simulink model "Simulink_MPC_LQR"  (R2025b)
settings: Solver=VariableStepAuto  StartTime=0.0  StopTime=50  RelTol=1e-3
InitFcn:
  | run("init.m");
StopFcn:
  | %run("video.m");
undefined symbols (not defined in the file or in its folder): robot_params
settings Model: Creator=Acer  LastModifiedBy=Acer

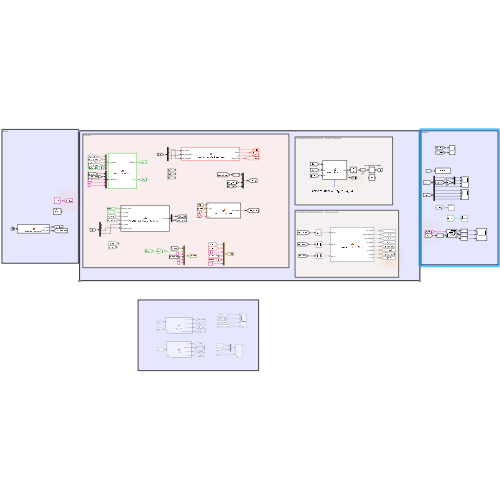
[thumbnail: Simulink's stored preview of the top-level diagram]
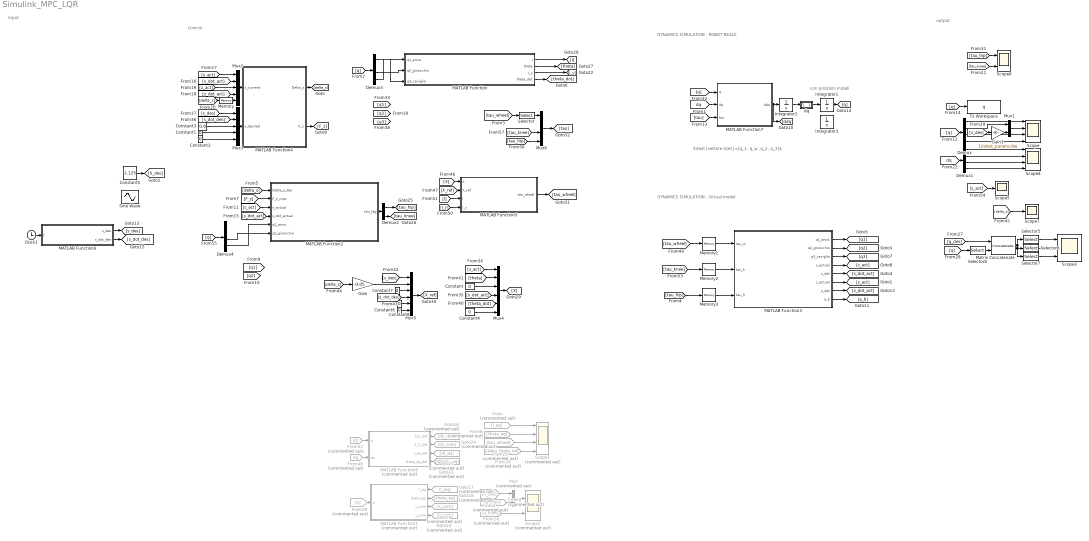
== system Simulink_MPC_LQR ==
  note: con posizioni iniziali
  note: input
  note: output
  note: DYNAMICS SIMULATION - ROBOT REALE
  note: $\text{vettore stati}=[q_1, q_w ,q_2, q_3]$
  note: Control
  note: DYNAMICS SIMULATION - Virtual model
  Clock1 : Clock
  Constant{,1..2,4,6..8} (7 alike) : Constant  Value=0
  Constant3 : Constant  Value=0.6
  Constant5 : Constant  Value=1.125
  Demux{,1,3..4} (4 alike) : Demux
  Demux2 : Demux  Outputs=2
  From : From  Commented=on  GotoTag=l_eq
  From23 : From  Commented=on  GotoTag=h_des
  From24 : From  Commented=on  GotoTag=s_com
  From25 : From  Commented=on  GotoTag=tau_wheel
  From26 : From  Commented=on  GotoTag=delta_theta_ref
  From39 : From  Commented=on  GotoTag=q
  From48 : From  Commented=on  GotoTag=dq  TagVisibility=global
  From52 : From  Commented=on  GotoTag=q
  From6 : From  Commented=on  GotoTag=theta_eq
  From8 : From  Commented=on  GotoTag=z_com
  Gain : Gain  Gain=-0.05
  Gain3 : Gain  Gain=1/robot_params.Rw
  Goto16 : Goto  Commented=on  GotoTag=ds_com
  Goto17 : Goto  Commented=on  GotoTag=l_eq
  Goto18 : Goto  Commented=on  GotoTag=theta_eq
  Goto19 : Goto  Commented=on  GotoTag=s_com
  Goto20 : Goto  Commented=on  GotoTag=z_com
  Goto21 : Goto  Commented=on  GotoTag=dl_eq
  Goto23 : Goto  Commented=on  GotoTag=dtheta_eq
  Goto24 : Goto  Commented=on  GotoTag=dz_com
  Integrator1 : Integrator  InitialCondition=[2.68;0;-2.34;1.23]
  Integrator2 : Integrator  InitialCondition=zeros(4,1)
  Integrator3 : Integrator  InitialCondition=[pi/2-0.1;zeros(3,1)]
  MATLAB Function : MATLAB Function  TreatAsAtomicUnit=on
  MATLAB Function1 : MATLAB Function  Commented=on  TreatAsAtomicUnit=on
  MATLAB Function2 : MATLAB Function  TreatAsAtomicUnit=on
  MATLAB Function3 : MATLAB Function  TreatAsAtomicUnit=on
  MATLAB Function4 : MATLAB Function  TreatAsAtomicUnit=on
  MATLAB Function5 : MATLAB Function  TreatAsAtomicUnit=on
  MATLAB Function6 : MATLAB Function  TreatAsAtomicUnit=on
  MATLAB Function7 : MATLAB Function  TreatAsAtomicUnit=on
  MATLAB Function8 : MATLAB Function  Commented=on  TreatAsAtomicUnit=on
  Matrix Concatenate : Concatenate  Mode=Multidimensional array  ConcatenateDimension=2
  Memory{,1..3} (4 alike) : Memory
  Mux : Mux  Commented=on  Inputs=2
  Mux1 : Mux  Inputs=2
  Mux2 : Mux  Inputs=5
  Mux3 : Mux  Inputs=5
  Mux4 : Mux  Inputs=6
  Mux5 : Mux  Inputs=6
  Mux6 : Mux
  Scope : Scope  NumInputPorts=4
      settings: ActiveDisplayString=4  Title=q3  ActiveDisplayYMinimum=-65.728095745464827  ActiveDisplayYMaximum=20.305803066962241
  Scope1 : Scope  Commented=on  NumInputPorts=4
      settings: ActiveDisplayString=4  Title=Delta_theta_ref  ActiveDisplayYMinimum=-0.047873246159911287  ActiveDisplayYMaximum=0.27907655031491813
  Scope2 : Scope  Commented=on  NumInputPorts=2
      settings: ActiveDisplayYMinimum=0.29186136198287116  ActiveDisplayYMaximum=1.3009042931130141  DataLoggingVariableName=ScopeData2
  Scope3 : Scope  NumInputPorts=3
      settings: ActiveDisplayYMinimum=2.02772604544463  ActiveDisplayYMaximum=2.8223539236982456  DataLoggingVariableName=ScopeData3
  Scope4 : Scope  NumInputPorts=4
      settings: Title=dq1  ActiveDisplayYMinimum=-1.1906100272021516  ActiveDisplayYMaximum=1.6920979215580041  DataLoggingVariableName=ScopeData4
  Scope5 : Scope
      settings: ActiveDisplayYMinimum=-44.629750975469719  ActiveDisplayYMaximum=5.655822114795205  DataLoggingVariableName=ScopeData5
  Scope7 : Scope
      settings: ActiveDisplayYMinimum=-0.6644623531131485  ActiveDisplayYMaximum=2.1105376468868529  DataLoggingVariableName=ScopeData7
  Scope8 : Scope  NumInputPorts=2
      settings: ActiveDisplayYMinimum=-6.3705206521435818  ActiveDisplayYMaximum=7.5706457083104626  DataLoggingVariableName=ScopeData8
  Selector : Selector  InputPortWidth=2  IndexOptions=Index vector (dialog)  Indices=1  OutputSizes=1
  Selector5 : Selector  NumberOfDimensions=2  InputPortWidth=3  IndexOptions=Index vector (dialog),Index vector (dialog)  Indices=[1],[1 2]  OutputSizes=1,1
  Selector6 : Selector  NumberOfDimensions=2  InputPortWidth=3  IndexOptions=Index vector (dialog),Index vector (dialog)  Indices=[2],[1 2]  OutputSizes=1,1
  Selector7 : Selector  NumberOfDimensions=2  InputPortWidth=3  IndexOptions=Index vector (dialog),Index vector (dialog)  Indices=[3],[1 2]  OutputSizes=1,1
  Selector8 : Selector  InputPortWidth=4  IndexOptions=Index vector (dialog)  Indices=[1 3 4]  OutputSizes=1
  Sine Wave : Sin  Amplitude=0.1  Bias=0.7  SampleTime=0
  To Workspace : ToWorkspace  VariableName=q  SaveFormat=Timeseries  SampleTime=-1
  dq : Subsystem
  wires:
  [tau] -> MATLAB Function7/3(tau)
  [q] -> MATLAB Function7/1(q)
  Integrator1/1 -> [q]
  MATLAB Function7/1(ddq) -> [ddq], Integrator2/1
  [dq] -> MATLAB Function7/2(dq)
  Integrator2/1 -> dq/1(In1)
  dq/1(Out1) -> Integrator1/1
  Demux/1 -> Scope/1
  Demux/3 -> Scope/3
  Demux/4 -> Scope/4
  [q] -> Demux/1
  [q] -> To Workspace/1
  MATLAB Function1/4(z_com) -> Goto20/1
  MATLAB Function8/2(Z_C_dot) -> Goto24/1
  MATLAB Function1/3(s_com) -> Goto19/1
  MATLAB Function8/4(theta_eq_dot) -> Goto23/1
  MATLAB Function1/1(l_eq) -> Goto17/1
  From52/1 -> MATLAB Function8/1(q)
  From39/1 -> MATLAB Function1/1(q)
  MATLAB Function1/2(theta_eq) -> Goto18/1
  MATLAB Function8/3(l_eq_dot) -> Goto21/1
  From48/1 -> MATLAB Function8/2(dq)
  MATLAB Function8/1(S_C_dot) -> Goto16/1
  From/1 -> Scope1/1
  From6/1 -> Scope1/2
  Constant5/1 -> [h_des]
  From8/1 -> Mux/2
  From23/1 -> Mux/1
  From24/1 -> Scope2/2
  Mux/1 -> Scope2/1
  [q_des] -> Matrix Concatenate/1
  Matrix Concatenate/1 -> Selector7/1, Selector6/1, Selector5/1
  Selector5/1 -> Scope3/1
  Selector6/1 -> Scope3/2
  Selector7/1 -> Scope3/3
  [q] -> Selector8/1
  Selector8/1 -> Matrix Concatenate/2
  From25/1 -> Scope1/3
  From26/1 -> Scope1/4
  Demux1/4 -> Scope4/4
  Demux1/3 -> Scope4/3
  Demux1/1 -> Scope4/1
  Demux1/2 -> Scope4/2
  [dq] -> Demux1/1
  [s_des] -> Gain3/1
  Mux1/1 -> Scope/2
  Demux/2 -> Mux1/1
  Gain3/1 -> Mux1/2
  MATLAB Function3/2(q2_ginocchio) -> [q2]
  MATLAB Function3/7(z_dot) -> [z_dot_act]
  Memory2/1 -> MATLAB Function3/2(tau_k)
  MATLAB Function3/3(q3_caviglia) -> [q3]
  [tau_knee] -> Memory2/1
  MATLAB Function3/8(a_b) -> [a_b]
  MATLAB Function3/1(q1_anca) -> [q1]
  MATLAB Function3/4(s_actual) -> [s_act]
  Memory3/1 -> MATLAB Function3/3(tau_h)
  [tau_hip] -> Memory3/1
  MATLAB Function3/5(s_dot) -> [s_dot_act]
  MATLAB Function3/6(z_actual) -> [z_act]
  Memory1/1 -> MATLAB Function3/1(tau_w)
  [tau_wheel] -> Memory1/1
  [s_dot_act] -> Mux2/2
  Memory/1 -> Mux2/5
  [z_dot_act] -> Mux2/4
  [s_act] -> Mux2/1
  [z_act] -> Mux2/3
  [delta_s] -> Memory/1
  Mux2/1 -> MATLAB Function4/1(x_current)
  MATLAB Function6/2(s_dot_des) -> [s_dot_des]
  Constant1/1 -> Mux3/4
  Constant3/1 -> Mux3/3
  Clock1/1 -> MATLAB Function6/1(t)
  MATLAB Function6/1(s_des) -> [s_des]
  Constant2/1 -> Mux3/5
  [s_des] -> Mux3/1
  [s_dot_des] -> Mux3/2
  Mux3/1 -> MATLAB Function4/2(x_desired)
  MATLAB Function4/1(Delta_s) -> [delta_s]
  MATLAB Function4/2(F_z) -> [F_z]
  [s_act] -> MATLAB Function2/3(s_actual)
  Demux4/3 -> MATLAB Function2/6(q2_ginocchio)
  [delta_s] -> MATLAB Function2/1(Delta_s_des)
  Demux4/4 -> MATLAB Function2/5(q1_anca)
  Demux2/1 -> [tau_hip]
  [F_z] -> MATLAB Function2/2(F_z_mpc)
  MATLAB Function2/1(tau_leg) -> Demux2/1
  [s_dot_act] -> MATLAB Function2/4(s_dot_actual)
  [tau_knee] -> Scope8/2
  [tau_hip] -> Scope8/1
  Demux2/2 -> [tau_knee]
  Demux3/3 -> MATLAB Function/2(q2_ginocchio)
  Demux3/1 -> MATLAB Function/3(q3_caviglia)
  Demux3/4 -> MATLAB Function/1(q1_anca)
  MATLAB Function/4(theta_dot) -> [theta_dot]
  MATLAB Function/3(I_y) -> [I_y]
  MATLAB Function/1(l) -> [l]
  MATLAB Function/2(theta) -> [theta]
  [s_act] -> Mux4/1
  [s_dot_act] -> Mux4/4
  [theta_dot] -> Mux4/5
  [theta] -> Mux4/2
  Constant/1 -> Mux4/3
  Constant4/1 -> Mux4/6
  Mux4/1 -> [X]
  Gain/1 -> Mux5/2
  [delta_s] -> Gain/1
  Mux5/1 -> [X_ref]
  [s_dot_des] -> Mux5/4
  [s_des] -> Mux5/1
  [delta_s] -> Scope7/1
  Constant7/1 -> Mux5/3
  Constant8/1 -> Mux5/5
  Constant6/1 -> Mux5/6
  [X] -> MATLAB Function5/1(X)
  [X_ref] -> MATLAB Function5/2(X_ref)
  [I_y] -> MATLAB Function5/4(I_y)
  [l] -> MATLAB Function5/3(l)
  MATLAB Function5/1(tau_wheel) -> [tau_wheel]
  [q] -> Demux3/1
  [s_act] -> Scope5/1
  [q] -> Demux4/1
  Mux6/1 -> [tau]
  [tau_knee] -> Mux6/3
  [tau_hip] -> Mux6/4
  [tau_wheel] -> Selector/1
  Selector/1 -> Mux6/1

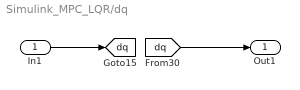
== system Simulink_MPC_LQR/dq ==
  In1 : Inport
  Out1 : Outport
  tag scope: dq=global
  wires:
  In1/1 -> [dq]
  [dq] -> Out1/1

== matlab function Simulink_MPC_LQR/MATLAB Function8 ==
  data: q input; dq input; S_C_dot output; Z_C_dot output; l_eq_dot output; theta_eq_dot output; robot_params parameter
function [S_C_dot, Z_C_dot, l_eq_dot, theta_eq_dot] = J_CoM(q,dq,robot_params)
    %#codegen
    % CALCOLA_VELOCITA_COM_SIMULINK Calcola le velocità del CoM e del pendolo 
    % equivalente (WIP) per l'utilizzo in Simulink.
    
    % --- 1. Estrazione Variabili di Stato ---
    q1 = q(1);
    q2 = q(3);
    q3 = q(4);
    
    % --- 2. Estrazione Parametri Robot ---
    l1 = robot_params.l1;
    l2 = robot_params.l2;
    l3 = robot_params.l3;
    
    m1 = robot_params.m1;
    m2 = robot_params.m2;
    m3 = robot_params.m3;
    m_upper = m1 + m2 + m3;
    
    % --- 3. Costanti Raggruppate per l'Analitica ---
    K1 = (m1 * (l1/2) + m2 * l1 + m3 * l1) / m_upper;
    K2 = (m2 * (l2/2) + m3 * l2) / m_upper;
    K3 = (m3 * (l3/2)) / m_upper;
    
    % --- 4. Ricalcolo Posizione CoM ---
    S_C = K1*cos(q1) + K2*cos(q1+q2) + K3*sin(q3);
    Z_C = K1*sin(q1) + K2*sin(q1+q2) + K3*cos(q3);
    
    % --- 5. Calcolo Jacobiano (J_CoM) ---
    % Preallocazione statica della matrice 2x4 per compatibilità C/C++
    J_CoM = zeros(2, 4);
    
   % --- 5. Calcolo Jacobiano (J_CoM) ---
    % Preallocazione statica della matrice 2x4 per compatibilità C/C++
    J_CoM = zeros(2, 4);
    
    % Derivate parziali di S_C (Prima Riga)
    J_CoM(1, 1) = -K1*sin(q1) - K2*sin(q1+q2); % <--- CORRETTO: indice (1,1) per dq1
    J_CoM(1, 3) = -K2*sin(q1+q2);              % <--- CORRETTO: indice (1,3) per dq2
    J_CoM(1, 4) =  K3*cos(q3);                 % <--- CORRETTO: indice (1,4) per dq3
    
    % Derivate parziali di Z_C (Seconda Riga)
    J_CoM(2, 1) =  K1*cos(q1) + K2*cos(q1+q2); % <--- CORRETTO: indice (2,1) per dq1
    J_CoM(2, 3) =  K2*cos(q1+q2);              % <--- CORRETTO: indice (2,3) per dq2
    J_CoM(2, 4) = -K3*sin(q3);                 % <--- CORRETTO: indice (2,4) per dq3
    % --- 6. Calcolo Velocità Cartesiane ---
    % V_C = [S_C_dot; Z_C_dot]
    V_C = J_CoM * dq;
    S_C_dot = V_C(1);
    Z_C_dot = V_C(2);
    
    % --- 7. Derivate del Pendolo Equivalente e Gestione Singolarità ---
    l_eq_sq = S_C^2 + Z_C^2;
    l_eq = sqrt(l_eq_sq);
    

        l_eq_dot = (S_C * S_C_dot + Z_C * Z_C_dot) / l_eq;
        theta_eq_dot = (S_C_dot * Z_C - S_C * Z_C_dot) / l_eq_sq;
   end

== matlab function Simulink_MPC_LQR/MATLAB Function ==
  settings: updateMethod=DISCRETE  sampleTime=0.001
  data: q1_anca input; l output; q2_ginocchio input; q3_caviglia input; theta output; I_y output; theta_dot output
function [l, theta, I_y, theta_dot] = calculate_equivalent_pendulum(q1_anca, q2_ginocchio, q3_caviglia)
    persistent theta_prev
    if isempty(theta_prev), theta_prev = 0; end
    dt = 0.001;

    % Somma degli angoli della catena
    theta = q1_anca + q2_ginocchio + q3_caviglia;
    theta_dot = (theta - theta_prev) / dt;
    theta_prev = theta;

    l = 2 * 0.45 * cos(q2_ginocchio / 2);
    if l < 0.1, l = 0.1; end
    m_b = 73.0;
    I_y = (1/3) * m_b * l^2;
end

== matlab function Simulink_MPC_LQR/MATLAB Function3 ==
  data: tau_w input; q1_anca output; tau_k input; tau_h input; q2_ginocchio output; q3_caviglia output; s_actual output; s_dot output; z_actual output; z_dot output; a_b output
function [q1_anca, q2_ginocchio, q3_caviglia, s_actual, s_dot, z_actual, z_dot, a_b] = Simulated_Robot_Plant(tau_w, tau_k, tau_h)
    q1_anca = 0.0; q2_ginocchio = 0.0; q3_caviglia = 0.0;
    s_actual = 0.0; s_dot = 0.0; z_actual = 0.0; z_dot = 0.0;
    a_b = zeros(2,1);

    persistent X_z X_wip
    if isempty(X_z)
        X_z = [0.6; 0];       
        X_wip = [0; 0; 0; 0]; 
    end
    dt = 0.001; g = 9.81; m_b = 73.0; r = 0.127; m_w = 3.5; I_w = 0.1; l = 0.45;

    %% 1. FISICA VERTICALE (Z)
    ratio = X_z(1) / (2*l);
    if ratio > 0.999, ratio = 0.999; elseif ratio < -0.999, ratio = -0.999; end
    q2_current = 2 * acos(ratio);
    
    J_z_knee = -l * sin(q2_current / 2);
    if abs(J_z_knee) < 0.05, J_z_knee = -0.05 * sign(q2_current + 1e-6); end
    
    F_z_applied = tau_k / J_z_knee; 
    z_ddot = (F_z_applied / m_b) - g;
    
    X_z(2) = X_z(2) + z_ddot * dt;
    X_z(1) = X_z(1) + X_z(2) * dt;
    
    % Blocchi fisici estremi per evitare decolli o sprofondamenti
    if X_z(1) < 0.2, X_z(1) = 0.2; X_z(2) = 0; end 
    if X_z(1) > 0.9, X_z(1) = 0.9; X_z(2) = 0; end 
    z_act = X_z(1);

    %% 2. FISICA DEL PENDOLO Orizzontale
    l_pend = z_act;
    if l_pend > 0.9, l_pend = 0.9; end 
    if l_pend < 0.1, l_pend = 0.1; end
    
    I_y = (1/3) * m_b * l_pend^2;

    D = 2*I_w*(I_y + m_b*l_pend^2) + (2*l_pend^2*m_b*m_w + I_y*(m_b + 2*m_w)*r^2);
    a1 = -(g * l_pend^2 * m_b^2 * r^2) / D;
    a2 =  (g * l_pend * m_b * (2*I_w + (m_b + 2*m_w)*r^2)) / D;
    b1 =  (r * (I_y + l_pend*m_b*(l_pend + r))) / D;
    b2 = -(2*I_w + r*(l_pend*m_b + (m_b + 2*m_w)*r)) / D;

    A_wip = [0 0 1 0; 0 0 0 1; 0 a1 0 0; 0 a2 0 0];
    B_wip = [0 0; 0 0; b1 b1; b2 b2];

    % LA CORREZIONE VITALE: Diamo ai motori la forza di bilanciare 73 kg!
    tau_w_lim = tau_w;
    limite = 1000; % Aumentato da 15 a 1000 Nm
    if tau_w_lim(1) > limite, tau_w_lim(1) = limite; end
    if tau_w_lim(1) < -limite, tau_w_lim(1) = -limite; end
    if tau_w_lim(2) > limite, tau_w_lim(2) = limite; end
    if tau_w_lim(2) < -limite, tau_w_lim(2) = -limite; end

    X_wip_dot = A_wip * X_wip + B_wip * tau_w_lim;
    X_wip = X_wip + X_wip_dot * dt;
    theta_vero = X_wip(2);

    %% 3. ASSEGNAZIONE GIUNTI (La tua convenzione perfetta)
    ratio_new = z_act / (2*l);
    if ratio_new > 0.999, ratio_new = 0.999; elseif ratio_new < -0.999, ratio_new = -0.999; end
    q2_ginocchio = 2 * acos(ratio_new);
    
    alpha = q2_ginocchio / 2;
    q3_caviglia = -alpha + theta_vero;
    q1_anca = -alpha;

    %% 4. ASSEGNAZIONE USCITE
    s_actual = X_wip(1);
    s_dot = X_wip(3);
    z_actual = z_act;
    z_dot = X_z(2);
    a_b = [X_wip_dot(3); z_ddot + g];
end

== matlab function Simulink_MPC_LQR/MATLAB Function6 ==
  data: t input; s_des output; s_dot_des output
function [s_des, s_dot_des] = Smooth_Trajectory(t)
    % PRE-ALLOCAZIONE PER IL CODER
    s_des = 0.0;
    s_dot_des = 0.0;
    
    % PARAMETRI DELLA TRAIETTORIA
    t_start = 0.0;       % Il robot inizia a muoversi a 2 secondi
    t_end = 5.0;         % Arriva a destinazione a 5 secondi (3 secondi di viaggio)
    s_final = 1.0;       % Destinazione orizzontale (1 metro)
    
    % LOGICA DEL MOVIMENTO
    if t <= t_start
        % Prima di partire, resta fermo
        s_des = 0.0;
        s_dot_des = 0.0;
        
    elseif t >= t_end
        % Arrivato a destinazione, fermati
        s_des = s_final;
        s_dot_des = 0.0;
        
    else
        % FASE DI MOTO: Polinomio Cubico (Minimum Jerk Trajectory)
        % Normalizziamo il tempo tra 0 e 1 per la durata del viaggio
        tau = (t - t_start) / (t_end - t_start);
        
        % Posizione (Profilo a "S" morbida)
        s_des = s_final * (3*tau^2 - 2*tau^3);
        
        % Velocità (Derivata della posizione, forma a campana)
        s_dot_des = s_final * (6*tau - 6*tau^2) / (t_end - t_start);
    end
end

== matlab function Simulink_MPC_LQR/MATLAB Function4 ==
  settings: updateMethod=DISCRETE  sampleTime=0.01
  data: x_current input; Delta_s output; x_desired input; F_z output
function [Delta_s,F_z] = MPC_Custom_QP(x_current, x_desired)
    % quadprog non è supportato nativamente per la code generation C
    coder.extrinsic('quadprog');
    coder.extrinsic('optimoptions');

    %% 1. Parametri e Discretizzazione
    m_b = 73.0; 
    g = 9.81;    
    
    h = x_current(3); 
    if h < 0.1
        h = 0.6;
    end
    
    dt = 0.01; 
    N = 40;     
    
    A_c = zeros(5,5);
    A_c(1,2) = 1;
    A_c(3,4) = 1;
    A_c(2,5) = g / h; 
    
    B_c = zeros(5,2);
    B_c(4,2) = 1 / m_b;
    B_c(5,1) = 1;
    
    A_d = eye(5) + A_c * dt;
    B_d = B_c * dt;

    %% 2. Pesi della Funzione di Costo
    S = diag([100, 10, 500, 50, 1]);
    W = diag([1, 0.01]);

    %% 3. Condensazione (Srotolamento) 
    nx = 5; nu = 2;
    P_x = zeros(nx*N, nx);
    P_u = zeros(nx*N, nu*N);

    A_power = eye(nx);
    for i = 1:N
        A_power = A_power * A_d;
        P_x((i-1)*nx+1 : i*nx, :) = A_power;
        for j = 1:i
            P_u((i-1)*nx+1 : i*nx, (j-1)*nu+1 : j*nu) = (A_d^(i-j)) * B_d;
        end
    end

    S_bar = kron(eye(N), S);
    W_bar = kron(eye(N), W);

    H = 2 * (P_u' * S_bar * P_u + W_bar);
    H = (H + H') / 2; % Garantisce simmetria perfetta
    
    X_ref = repmat(x_desired, N, 1);
    f = 2 * P_u' * S_bar * (P_x * x_current - X_ref);

    %% 4. Vincoli Fisici
    F_min = -1500; % Permette di frenare!
    F_max = 1500;
    
    LB = zeros(nu*N, 1);
    UB = zeros(nu*N, 1);
    
    for i = 1:N
        LB((i-1)*nu+1) = -2.0; 
        UB((i-1)*nu+1) = 2.0;
        
        LB((i-1)*nu+2) = F_min; 
        UB((i-1)*nu+2) = F_max;
    end

    %% 5. Risoluzione QP (CORRETTA)
    % Pre-allocazione per Simulink Coder
    U_opt_calc = zeros(nu*N, 1);
    fval = 0.0;
    exitflag = 0.0;
    
    % Algoritmo robusto di default
    options = optimoptions('quadprog', 'Display', 'off');
    
    % LA CORREZIONE: Aggiunto "fval" per non sballare "exitflag"!
    [U_opt_calc, fval, exitflag] = quadprog(H, f, [], [], [], [], LB, UB, [], options);

    if exitflag > 0
        U_opt = U_opt_calc;
    else
        % Se fallisce davvero, eroga 0 extra, ma il VMC ci terrà in piedi col peso base
        U_opt = zeros(nu*N, 1);
    end

    %% 6. Estrazione Input Ottimo
    Delta_s_dot_opt = U_opt(1);
    F_z = U_opt(2); % FINALMENTE SARA' DIVERSO DA ZERO!

    Delta_s = x_current(5) + Delta_s_dot_opt * dt;
end

== matlab function Simulink_MPC_LQR/MATLAB Function2 ==
  data: Delta_s_des input; tau_leg output; F_z_mpc input; s_actual input; s_dot_actual input; q1_anca input; q2_ginocchio input
function tau_leg = VMC_Task_Space_Controller(Delta_s_des, F_z_mpc, s_actual, s_dot_actual, q1_anca, q2_ginocchio)
    tau_leg = zeros(2, 1);
    l = 0.45; m_tot = 73.0; g = 9.81;
    
    % Jacobiano lineare per il ginocchio
    J_z_knee = -l * sin(q2_ginocchio / 2);
    if abs(J_z_knee) < 0.05, J_z_knee = -0.05 * sign(q2_ginocchio + 1e-6); end
    
    F_z_totale = F_z_mpc + (m_tot * g);
    
    % Il ginocchio assorbe la spinta. L'anca sta a 0 (passiva)
    tau_k = J_z_knee * F_z_totale;
Kp_h = 200;  % da tarare
% Delta_s_actual: lo spostamento orizzontale attuale del baricentro
% (puoi calcolarlo dalla geometria delle gambe, es. l*sin(theta_gamba))
Delta_s_actual = s_actual;  % oppure una stima geometrica più precisa se disponibile
tau_h = Kp_h * (Delta_s_des - Delta_s_actual);    
    tau_leg = [tau_k; tau_h];
end

== matlab function Simulink_MPC_LQR/MATLAB Function5 ==
  data: X input; tau_wheel output; X_ref input; l input; I_y input
function tau_wheel = TV_LQR_Controller(X, X_ref, l, I_y)
    % X: Stato attuale [s; theta; phi; s_dot; theta_dot; phi_dot] (6x1)
    % X_ref: Stato target desiderato [s_ref; theta_ref; phi_ref; 0; 0; 0] (6x1)
    % l: Lunghezza attuale del pendolo equivalente [m]
    % I_y: Inerzia attuale del corpo superiore [kg*m^2]
    
    % Per usare la funzione lqr() di MATLAB all'interno di Simulink, 
    % dobbiamo dichiararla come estrinseca.
    coder.extrinsic('lqr');
    
    % 1. Richiamo Parametri Fisici
    m_w = 3.5;       % Massa ruota
    I_w = 0.1;       % Inerzia ruota
    r   = 0.127;     % Raggio ruota
    d   = 0.63;      % Distanza ruote
    m_b = 73.0;      % Massa corpo superiore
    I_z = 3.3;       % Inerzia torso asse z
    g   = 9.81;      % Gravità
    
    % 2. Calcolo dei Coefficienti della Dinamica (Eq. 14)
    % Denominatore comune per a1, a2, b1, b2
    D = 2*I_w*(I_y + m_b*l^2) + (2*l^2*m_b*m_w + I_y*(m_b + 2*m_w)*r^2);
    
    a1 = -(g * l^2 * m_b^2 * r^2) / D;
    a2 =  (g * l * m_b * (2*I_w + (m_b + 2*m_w)*r^2)) / D;
    
    b1 =  (r * (I_y + l*m_b*(l + r))) / D;
    b2 = -(2*I_w + r*(l*m_b + (m_b + 2*m_w)*r)) / D;
    
    % Coefficiente disaccoppiato per lo steering (imbardata)
    b3 =  (d * r) / (2*I_z*r^2 + d^2*(I_w + m_w*r^2));
    
    % 3. Costruzione Matrici di Stato A(l) e Input B(l) (Eq. 12, Eq. 13)
    A = zeros(6, 6);
    A(1, 4) = 1; 
    A(2, 5) = 1; 
    A(3, 6) = 1;
    A(4, 2) = a1;
    A(5, 2) = a2;
    
    B = zeros(6, 2);
    B(4, 1) = b1;  B(4, 2) = b1;
    B(5, 1) = b2;  B(5, 2) = b2;
    B(6, 1) = b3;  B(6, 2) = -b3;
    
    % 4. Definizione Matrici di Peso Q e R (Tuning LQR)
    % Questi valori determinano l'aggressività del controllore. 
    % Possono essere trasformati in input del blocco per un tuning rapido.
    % 4. Definizione Matrici di Peso Q e R (Tuning Soft)
    % Pesi drasticamente ridotti per evitare instabilità con il ritardo discreto
% Aumenta il peso sugli angoli (q1, q2) per evitare che saturino
    Q = diag([50, 50, 100, 50, 10, 1]);
    R = diag([1, 1]) * 0.5;         % Penalizziamo maggiormente l'uso eccessivo dei motori
    
    % 5. Risoluzione LQR e Calcolo Input
    % Inizializza K per la Code Generation di Simulink
    K = zeros(2, 6); 
    
    % Calcola la matrice dei guadagni ottimali K
    K = lqr(A, B, Q, R);
    
    % Errore di stato (tilde_X)
    X_tilde = X - X_ref;
    
    % Legge di controllo finale (Eq. 16): U = [tau_l; tau_r]
    tau_wheel = -K * X_tilde; 
end

== matlab function Simulink_MPC_LQR/MATLAB Function1 ==
  data: q input size=4; l_eq output; theta_eq output; s_com output; z_com output; robot_params parameter
function [l_eq,theta_eq, s_com, z_com] = CoM(q,robot_params)

[l_eq,theta_eq, s_com, z_com] = calcola_CoM_equivalente(q, robot_params);

end

== matlab function Simulink_MPC_LQR/MATLAB Function7 ==
  data: q input; ddq output size=4; dq input; tau input
function ddq =  whole_robot_2D(q, dq, tau)
    % tau è il vettore delle coppie/forze generalizzate in ingresso (4x1)
    
    [M, CdQ, G] = calc_dynamics(q, dq);

    %% equazione del moto: M*ddq + C*dq + G = tau
    % In MATLAB/Simulink si usa l'operatore mldivide (\) per invertire M in modo robusto
    ddq = M \ (tau - CdQ - G);
end
